simulink model "subsistem"  (Simulink 6.0)
settings: Solver=ode45  StartTime=0.0  StopTime=10.0  RelTol=1e-3
libraries: fuzblock x1
settings Model: LastModifiedBy=student

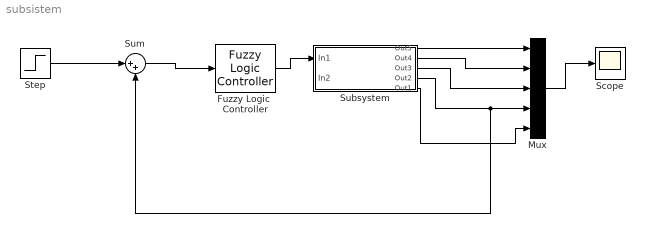
== system subsistem ==
  Fuzzy Logic  Controller : fuzblock/Fuzzy Logic  Controller  fis=regP
  Mux : Mux  Inputs=5
  Scope : Scope
  Step : Step  SampleTime=0
  Subsystem : Subsystem
  Sum : Sum  Inputs=|++
  wires:
  Step/1 -> Sum/1
  Fuzzy Logic  Controller/1 -> Subsystem/1(In1)
  Sum/1 -> Fuzzy Logic  Controller/1
  Subsystem/1(Out5) -> Mux/1
  Subsystem/2(Out4) -> Mux/2
  Subsystem/3(Out3) -> Mux/3
  Subsystem/4(Out2) -> Mux/4, Sum/2
  Subsystem/5(Out1) -> Mux/5
  Mux/1 -> Scope/1

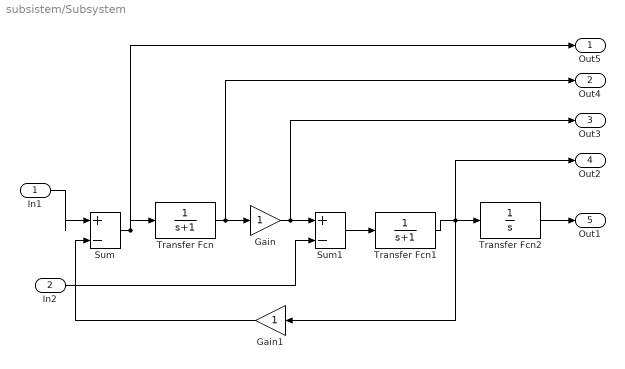
== system subsistem/Subsystem ==
  In1 : Inport  Port=1  LatchInput=off
  In2 : Inport  Port=2  LatchInput=off
  Gain : Gain
  Gain1 : Gain  Orientation=left
  Sum : Sum  Inputs=|+-
  Sum1 : Sum  Inputs=|+-
  Transfer Fcn : TransferFcn  Denominator=[1 1]
  Transfer Fcn1 : TransferFcn  Denominator=[1 1]
  Transfer Fcn2 : TransferFcn  Denominator=[1 0]
  Out5 : Outport
  Out4 : Outport  Port=2
  Out3 : Outport  Port=3
  Out2 : Outport  Port=4
  Out1 : Outport  Port=5
  wires:
  Sum/1 -> Transfer Fcn/1, Out5/1
  Transfer Fcn/1 -> Gain/1, Out4/1
  Gain/1 -> Sum1/1, Out3/1
  Sum1/1 -> Transfer Fcn1/1
  Transfer Fcn1/1 -> Transfer Fcn2/1, Gain1/1, Out2/1
  In2/1 -> Sum1/2
  Gain1/1 -> Sum/2
  Transfer Fcn2/1 -> Out1/1
  In1/1 -> Sum/1
